simulink model "TD_PITCH"  (R2019b)
settings: Solver=VariableStepAuto  StartTime=0.0  StopTime=10.0  RelTol=1e-3
undefined symbols (not defined in the file): Dm, Dt, F_limit_pitch, g, Jp, k_pitch, Mb
settings Model: Creator=lbend  LastModifiedBy=lbend

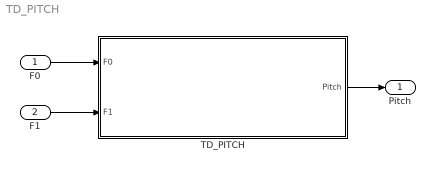
== system TD_PITCH ==
  F0 : Inport
  "F1 " : Inport  Port=2
  TD_PITCH : Subsystem
  Pitch : Outport
  wires:
  F0/1 -> TD_PITCH/1(F0)
  "F1 "/1 -> TD_PITCH/2("F1 ")
  TD_PITCH/1(Pitch) -> Pitch/1

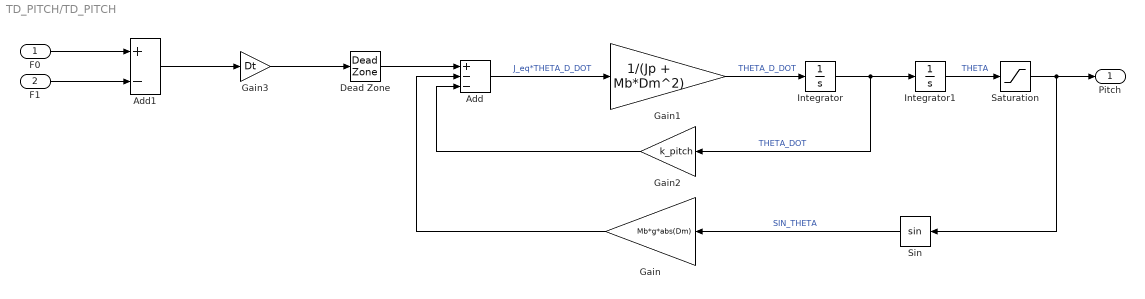
== system TD_PITCH/TD_PITCH ==
  F0 : Inport
  "F1 " : Inport  Port=2
  Add : Sum  Inputs=+--
  Add1 : Sum  Inputs=+-
  Dead Zone : DeadZone  LowerValue=F_limit_pitch/2  UpperValue=F_limit_pitch/2  SaturateOnIntegerOverflow=on
  Gain : Gain  Gain=Mb*g*abs(Dm)
  Gain1 : Gain  Gain=1/(Jp + Mb*Dm^2)
  Gain2 : Gain  Gain=k_pitch
  Gain3 : Gain  Gain=Dt
  Integrator : Integrator
  Integrator1 : Integrator
  Saturation : Saturate  UpperLimit=0.93  LowerLimit=-0.93
  Sin : Trigonometry
  Pitch : Outport
  wires:
  Gain2/1 -> Add/3
  Saturation/1 -> Sin/1, Pitch/1
  Sin/1 -> Gain/1  "SIN_THETA"
  Integrator/1 -> Integrator1/1, Gain2/1  "THETA_DOT"
  Add/1 -> Gain1/1  "J_eq*THETA_D_DOT"
  Add1/1 -> Gain3/1
  Gain1/1 -> Integrator/1  "THETA_D_DOT"
  Gain/1 -> Add/2
  "F1 "/1 -> Add1/2
  Integrator1/1 -> Saturation/1  "THETA"
  F0/1 -> Add1/1
  Gain3/1 -> Dead Zone/1
  Dead Zone/1 -> Add/1
